simulink library "EV_ePWT"  (R2019b)
settings: Solver=VariableStepAuto  StartTime=0.0  StopTime=10.0  RelTol=1e-3
undefined symbols (not defined in the file): BTR, DiscIntNeverNeededParam, INV
libraries: simulink x1
(part 1 of 2)
Description:
  | User defined library for EV
settings Model: Creator=francesco.mantuano  LastModifiedBy=matteo.paganini

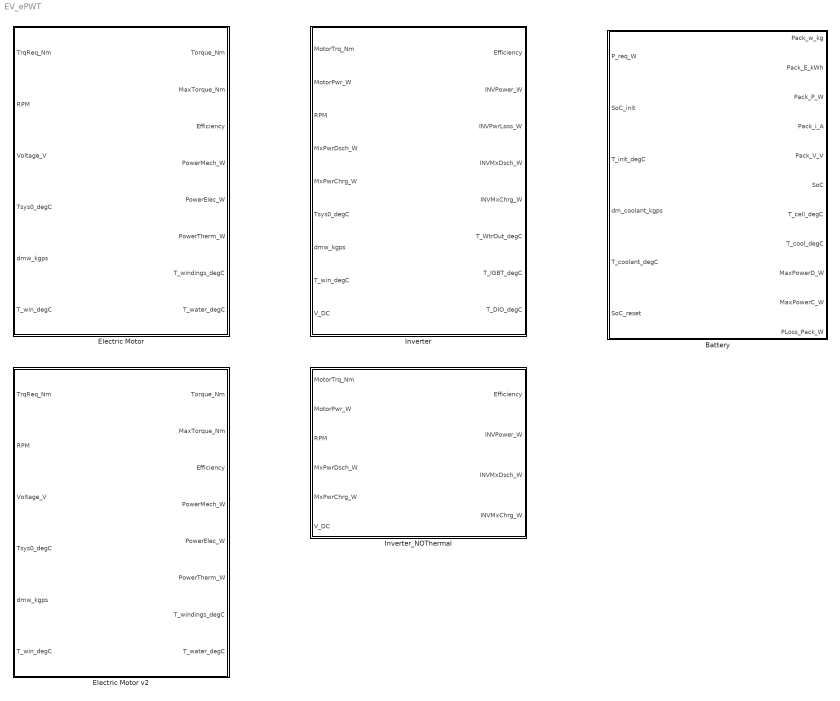
== system EV_ePWT ==
  Battery : Subsystem  mask(Battery 1RC){n_series=BTR.cell_p.n_series, n_parallel=BTR.cell_p.n_parallel, weight_ratio=0.7, C_cell_Ah=BTR.cell_p.capacity_nom, V_nominal=BTR.cell_p.voltage_nom, R_contact=0, V_low=BTR.cell_p.Vmin, V_up=BTR.cell_p.Vmax, R_th_KpW=BTR.cell_p.R_th, c_th=BTR.cell_p.c_th, weight=BTR.cell_p.weight, VoC_map=BTR.cell_p.VOC, VoC_SoC_bp=BTR.cell_p.SOC_bp_VOC, VoC_Temp_bp=BTR.cell_p.Temp_bp_VOC, VoC_C_bp=BTR.cell_p.C_bp, R0_map=BTR.cell_p.R0, R0_SoC_bp=BTR.cell_p.SOC_bp, R0_Temp_bp=BTR.cell_p.Temp_bp, R0_i_bp=BTR.cell_p.I_bp, R0_C_bp=BTR.cell_p.C_bp, R1_map=BTR.cell_p.R1, R1_SoC_bp=BTR.cell_p.SOC_bp, R1_Temp_bp=BTR.cell_p.Temp_bp, R1_i_bp=BTR.cell_p.I_bp, R1_C_bp=BTR.cell_p.C_bp, tau1_map=BTR.cell_p.tau, tau1_SoC_bp=BTR.cell_p.SOC_bp, tau1_Temp_bp=BTR.cell_p.Temp_bp, tau1_i_bp=BTR.cell_p.I_bp, tau1_C_bp=BTR.cell_p.C_bp, Limit_temp_bp=[-30 -10 0 55 57 58], Limit_map=[0 0.2 1 1 0.2 0], max_peak_crate=5, max_crate=2, peak_time=10}
      mask prompts: n_series "number of series"; n_parallel "number of parallel"; weight_ratio "cells/total weight ratio [-]"; C_cell_Ah "cell capacity [Ah]"; V_nominal "Nominal voltage [V]"; R_contact "R_contact [ohm]"; V_low "Voltage lower limit [V]"; V_up "Voltage upper limit [V]"; R_th_KpW "Thermal resistance [K/W]"; c_th "Specific heat capacity [J/(kgK)]"; weight "Cell weight [kg]"; VoC_map "Voltage map [V]"; VoC_SoC_bp "SoC breakpoints [-]"; VoC_Temp_bp "Temp breakpoints [degC]"; VoC_C_bp "C breakpoints [Ah]"; R0_map "R0 map [ohm]"; R0_SoC_bp "SoC breakpoints [-]"; R0_Temp_bp "Temp breakpoints [degC]"; R0_i_bp "i_cell breakpoints [A]"; R0_C_bp "C breakpoints [Ah]"; R1_map "R1 map [ohm]"; R1_SoC_bp "SoC breakpoints [-]"; R1_Temp_bp "Temp breakpoints [degC]"; R1_i_bp "i_cell breakpoints [A]"; R1_C_bp "C breakpoints [Ah]"; tau1_map "tau1 map [s]"; tau1_SoC_bp "SoC breakpoints [-]"; tau1_Temp_bp "Temp breakpoints [degC]"; tau1_i_bp "i_cell breakpoints [A]"; tau1_C_bp "C breakpoints [Ah]"; Limit_temp_bp "Limit Temp breakipoints [degC]"; Limit_map "Limit map [-]"; max_peak_crate "Max peak C-rate [1/h]"; max_crate "Max continuous C-rate [1/h]"; peak_time "C-rate peak time [s]"
      mask help:
      | 1RC battery model with simple BMS for c-rate, temperature and voltage limitations.
      | Includes simple thermal model and batery pack weights estimation
      mask DialogControl Container2 Prompt: Inputs description
      mask DialogControl DescTextVar Prompt: - P_req_W: power requested to battery [W] (negative is charge)
      mask DialogControl DescTextVar2 Prompt: - SoC_init: State of Charge initialization [-] (0 < SoC_init < 1)
      mask DialogControl DescTextVar3 Prompt: - T_init_degC: Cell temperature initialization [degC]
      mask DialogControl DescTextVar4 Prompt: - SoC_reset: reset of SoC (reset with falling to 0)
      mask DialogControl Container3 Prompt: Battery parameters
      mask DialogControl Container15 Prompt: Inputs
      mask DialogControl Container16 Prompt: Pack
      mask DialogControl Container17 Prompt: cell
      mask DialogControl Container20 Prompt: Thermals
      mask DialogControl Container9 Prompt: Cell properties
      mask DialogControl Container10 Prompt: Voltage f(SoC,Temp,C)
      mask DialogControl Container11 Prompt: R0 f(SoC,Temp,i_cell,C)
      mask DialogControl Container12 Prompt: R1 f(SoC,Temp,i_cell,C)
      mask DialogControl Container13 Prompt: tau1 f(SoC,Temp,i_cell,C)
      mask DialogControl Container18 Prompt: SOF
      mask DialogControl Container22 Prompt: Temperature limitation
      mask DialogControl Container23 Prompt: C-rate limitation
  Electric Motor : Subsystem  mask(Motor){Mass_w=1, cp_w=385, Mass_s=1, cp_s=385, ThrmRtos=0.005, ThrmRtow=0.005, MaxT=180, RPM_bp1=0, voltage_bp=0, Torque_map=0, RPM_bp2=0, torque_bp=0, temp_bp=0, Efficiency_map=0}
      mask prompts: Mass_w "Windings Mass [kg]"; cp_w "Windings cp [J/(kg*K)]"; Mass_s "Stator Mass [kg]"; cp_s "Stator av. cp [J/(kg*K)]"; ThrmRtos "Thermal resistance 1 [K/W]"; ThrmRtow "Thermal resistance 2 [K/W]"; MaxT "Max temperature [degC] allowed"; RPM_bp1 "RPM breakpoints"; voltage_bp "Voltage [V] breakpoints"; Torque_map "Torque map [Nm]"; RPM_bp2 "RPM breakpoints"; torque_bp "Torque [Nm] breakpoints"; temp_bp "Temperature [degC] breakpoints"; Efficiency_map "Efficiency map [-]"
      mask help:
      | The Motor block is a map based block. It has as output the limited torque, power and efficiency.
      | It also includes a thermal model that outputs the motor and cooling liquid temperature.
      |
      | The inputs required are the torque(RPM, V) and efficiency(RPM, Trq, Temp) maps. The derating is thermal; the windings temperature is calculated taking into account the thermal capacity [J/K] and the thermal resistance [K/W]. "Thermal resistance 1" is the one between the windings and the stator, "Thermal resistance 2" is the one between the stator and the liquid cooling (constant with massflow).
      mask DialogControl Container2 Prompt: Input signals description
      mask DialogControl DescTextVar Prompt: - TrqReq_Nm: torque requested [Nm]
      mask DialogControl Control3 Prompt: - RPM: actual RPM of the motor
      mask DialogControl Control6 Prompt: - Voltage_V: voltage of the Inverter [V]
      mask DialogControl Control4 Prompt: - Tsys0_degC: initial temperature of the system [degC]
      mask DialogControl Control5 Prompt: - dmw_kgps: mass flow of the cooling liquid [kg/s]
      mask DialogControl Control7 Prompt: - T_win_degC: liquid cooling inlet temperature [degC]
      mask DialogControl Container3 Prompt: Motor parameters
      mask DialogControl Container9 Prompt: Constants
      mask DialogControl Container5 Prompt: Torque map
      mask DialogControl Container5_copy Prompt: Efficiency map
  Electric Motor v2 : Subsystem  mask(Motor){Mass_w=1, cp_w=385, Mass_s=1, cp_s=385, ThrmRtos=0.005, MaxT=180, RPM_bp1=0, voltage_bp=0, Torque_map=0, RPM_bp2=0, torque_bp=0, temp_bp=0, Efficiency_map=0, PL_torque_bp=-250:50:250, PL_RPM_bp=1000:1000:15000, PL_V_bp=450:100:750, PL_map=ones(11,15,4)*200, D_h=13.33e-3, A_n=2e-4, lpm_tar=10, R_tar=0.0154, thermal_mode=from efficiency maps}
      mask prompts: Mass_w "Windings Mass [kg]"; cp_w "Windings cp [J/(kg*K)]"; Mass_s "Stator Mass [kg]"; cp_s "Stator av. cp [J/(kg*K)]"; ThrmRtos "Thermal resistance 1 [K/W]"; MaxT "Max temperature [degC] allowed"; RPM_bp1 "RPM breakpoints"; voltage_bp "Voltage [V] breakpoints"; Torque_map "Torque map [Nm]"; RPM_bp2 "RPM breakpoints"; torque_bp "Torque [Nm] breakpoints"; temp_bp "Temperature [degC] breakpoints"; Efficiency_map "Efficiency map [-]"; PL_torque_bp "Torque [Nm] breakpoints"; PL_RPM_bp "RPM breakpoints"; PL_V_bp "V_DC [V] breakpoints"; PL_map "Power losses map [W]"; D_h "Hydraulic diameter [m]"; A_n "Normal surface [sm]"; lpm_tar "Refernce flowrate [lpm]"; R_tar "Target R_th @lpm_ref"; thermal_mode "Thermal losses calculation"
      mask help:
      | The Motor block is a map based block. It has as output the limited torque, power and efficiency.
      | It also includes a thermal model that outputs the motor and cooling liquid temperature.
      |
      | The inputs required are the torque(RPM, V) and efficiency(RPM, Trq, Temp) maps. The derating is thermal; the windings temperature is calculated taking into account the thermal capacity [J/K] and the thermal resistance [K/W]. "Thermal resistance 1" is the one between the windings and the stator, the thermal resistance between the stator and the liquid cooling is calculated with Dittus-Boelter correlation (open block to inspect the formula).
      mask TypeOptions thermal_mode: from efficiency maps | from power losses maps
      mask DialogControl Container2 Prompt: Input signals description
      mask DialogControl DescTextVar Prompt: - TrqReq_Nm: torque requested [Nm]
      mask DialogControl Control3 Prompt: - RPM: actual RPM of the motor
      mask DialogControl Control6 Prompt: - Voltage_V: voltage of the Inverter [V]
      mask DialogControl Control4 Prompt: - Tsys0_degC: initial temperature of the system [degC]
      mask DialogControl Control5 Prompt: - dmw_kgps: mass flow of the cooling liquid [kg/s]
      mask DialogControl Control7 Prompt: - T_win_degC: liquid cooling inlet temperature [degC]
      mask DialogControl Container3 Prompt: Motor parameters
      mask DialogControl Container9 Prompt: Constants
      mask DialogControl Container5 Prompt: Torque map
      mask DialogControl Container5_copy Prompt: Efficiency map
      mask DialogControl Container5_copy_copy_copy Prompt: Power losses map
      mask DialogControl Container5_copy_copy Prompt: Cooling (geometrical data)
  Inverter : Subsystem  mask(Inverter){C_IGBT=45, R_IGBT=0.038, C_DIO=10, R_DIO=0.070, C_HS=200, R_TIM=0.021, cp_cool=3140, n_poles=6, V_DC_ref=730, RPM_bp=1000:1000:15000, torque_bp=-250:50:250, Efficiency_map=ones(15,11)*0.95, PL_torque_bp=-250:50:250, PL_RPM_bp=1000:1000:15000, PL_V_bp=450:100:750, PL_map=ones(11,15,4)*200, thermal_mode=from efficiency maps}
      mask prompts: C_IGBT "Heat capacity [J/K]"; R_IGBT "Thermal resistance [K/W]"; C_DIO "Heat capacity [J/K]"; R_DIO "Thermal resistance [K/W]"; C_HS "HS Heat capacity [J/K]"; R_TIM "TIM Thermal resistance [K/W]"; cp_cool "cp water-glycol 50-50"; n_poles "number of pole pairs"; RPM_bp "RPM breakpoints"; torque_bp "Torque [Nm] breakpoints"; Efficiency_map "Efficiency map [-]"; PL_torque_bp "Torque [Nm] breakpoints"; PL_RPM_bp "RPM breakpoints"; PL_V_bp "V_DC [V] breakpoints"; PL_map "Power losses map [W]"; thermal_mode "Thermal losses calculation"
      mask help:
      | The Inverter block is a map based block. It has as output the efficiency, power and max deliverable power.
      | It also includes a thermal model that outputs the IGBT, Diode and cooling liquid temperature.
      mask TypeOptions thermal_mode: from efficiency maps | from power losses maps
      mask DialogControl Container2 Prompt: Inputs description
      mask DialogControl DescTextVar Prompt: - MotorTrq_Nm: motor torque [Nm]
      mask DialogControl DescTextVar_copy Prompt: - MotorPwr_W: motor electric power [W]
      mask DialogControl Control3 Prompt: - RPM: actual RPM of the motor
      mask DialogControl Control6 Prompt: - MxPwrDsch_W: max DC discharge deliverable power [W]
      mask DialogControl Control6_copy Prompt: - MxPwrChrg_W: max DC charge deliverable power [W]
      mask DialogControl Control4 Prompt: - Tsys0_degC: initial temperature of the system [degC]
      mask DialogControl Control5 Prompt: - dmw_kgps: mass flow of the cooling liquid [kg/s]
      mask DialogControl Control7 Prompt: - T_win_degC: liquid cooling inlet temperature [degC]
      mask DialogControl Container3 Prompt: Inverter parameters
      mask DialogControl Container9 Prompt: Constants
      mask DialogControl Container10 Prompt: IGBT
      mask DialogControl Container10_copy Prompt: DIODE
      mask DialogControl Container10_copy_copy Prompt: OTHER
      mask DialogControl Container5_copy Prompt: Efficiency map
      mask DialogControl Container5_copy_copy Prompt: Power losses map
  Inverter_NOThermal : Subsystem  mask(Inverter){RPM_bp=INV.Front.bp_RPM_Mtr, torque_bp=INV.Front.bp_Torque_Nm_Mtr, Efficiency_map=INV.Front.Eff_Table_r}
      mask prompts: RPM_bp "RPM breakpoints"; torque_bp "Torque [Nm] breakpoints"; Efficiency_map "Efficiency map [-]"
      mask help: The Inverter block is a map based block. It has as output the efficiency, power and max deliverable power.
      mask DialogControl Container2 Prompt: Inputs description
      mask DialogControl DescTextVar Prompt: - MotorTrq_Nm: motor torque [Nm]
      mask DialogControl DescTextVar_copy Prompt: - MotorPwr_W: motor electric power [W]
      mask DialogControl Control3 Prompt: - RPM: actual RPM of the motor
      mask DialogControl Control6 Prompt: - MxPwrDsch_W: max DC discharge deliverable power [W]
      mask DialogControl Control6_copy Prompt: - MxPwrChrg_W: max DC charge deliverable power [W]
      mask DialogControl Container3 Prompt: Inverter parameters
      mask DialogControl Container5_copy Prompt: Efficiency map

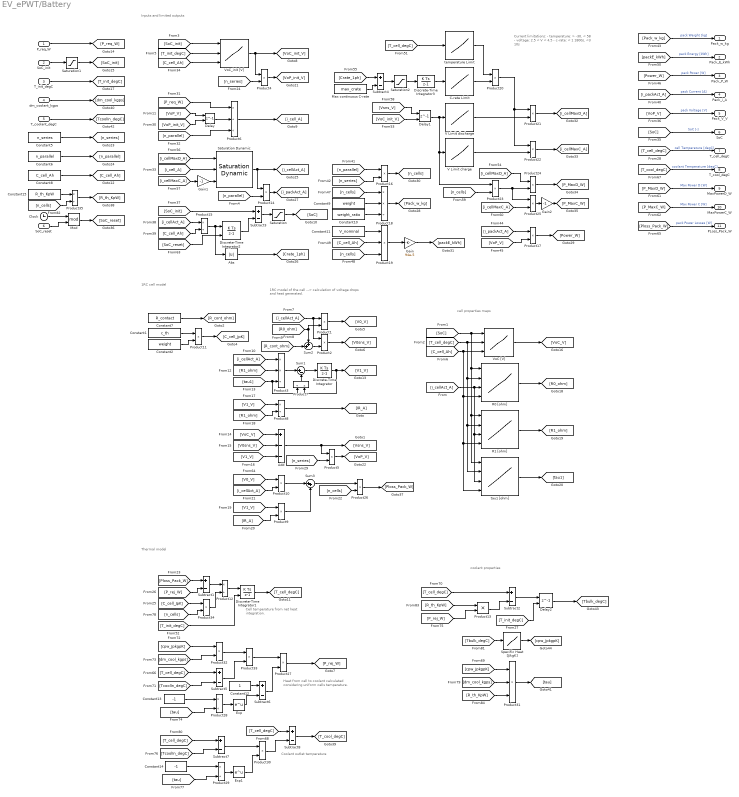
== system EV_ePWT/Battery ==
  note: 1RC model of the cell --> calculation of voltage drops and heat generated.
  note: cell properties maps
  note: Current limitations:
      | - temperature: > -30, < 58
      | - voltage: 2.5 < V < 4.5
      | - c-rate: < 1 1800s, <3 10s
  note: Inputs and limited outputs
  note: 1RC cell model
  note: Heat from cell to coolant calculated considering uniform cells temperature.
  note: Thermal model
  note: Cell temperature from net heat integration.
  note: Coolant outlet temperature
  note: coolant properties
  P_req_W : Inport
  SoC_init : Inport  Port=2
  T_init_degC : Inport  Port=3
  dm_coolant_kgps : Inport  Port=4
  T_coolant_degC : Inport  Port=5
  SoC_reset : Inport  Port=6
  Abs : Abs
  Add : Sum  Inputs=+--
  C-rate Limit : Lookup_n-D  NumberOfTableDimensions=1  BreakpointsForDimension1=[0 peak_time 60]  BreakpointsForDimension2=BTR.cell_p.Temp_bp_VOC  BreakpointsForDimension3=BTR.cell_p.C_bp  Table=[max_peak_crate max_peak_crate max_crate]*C_cell_Ah  ExtrapMethod=Clip  InternalRulePriority=Speed  RndMeth=Simplest  InputSameDT=on
  Clock : Clock
  Constant1 : Constant  Value=c_th
  Constant10 : Constant  Value=weight_ratio
  Constant11 : Constant  Value=V_nominal
  Constant12 : Constant
  Constant13 : Constant  Value=-1
  Constant14 : Constant  Value=-1
  Constant15 : Constant  Value=R_th_KpW
  Constant2 : Constant  Value=weight
  Constant5 : Constant  Value=n_series
  Constant6 : Constant  Value=n_parallel
  Constant7 : Constant  Value=R_contact
  Constant8 : Constant  Value=C_cell_Ah
  Constant9 : Constant  Value=weight
  Delay : Delay  DelayLength=1  InitialConditionSource=Input port
      settings: InputPortMap=u0,p4
  Delay1 : Delay  DelayLength=1  InitialConditionSource=Input port
      settings: InputPortMap=u0,p4
  Delay2 : Delay  DelayLength=1  InitialConditionSource=Input port
      settings: InputPortMap=u0,p4
  Discrete-Time Integrator : DiscreteIntegrator  SampleTime=-1  ICPrevOutput=DiscIntNeverNeededParam  ICPrevScaledInput=DiscIntNeverNeededParam
  Discrete-Time Integrator1 : DiscreteIntegrator  InitialConditionSource=external  SampleTime=-1  ICPrevOutput=DiscIntNeverNeededParam  ICPrevScaledInput=DiscIntNeverNeededParam
  Discrete-Time Integrator2 : DiscreteIntegrator  gainval=1/3600  ExternalReset=falling  SampleTime=-1  UpperSaturationLimit=1  LowerSaturationLimit=0  ICPrevOutput=DiscIntNeverNeededParam  ICPrevScaledInput=DiscIntNeverNeededParam
  Discrete-Time Integrator3 : DiscreteIntegrator  gainval=1  SampleTime=-1  LimitOutput=on  LowerSaturationLimit=0  ICPrevOutput=DiscIntNeverNeededParam  ICPrevScaledInput=DiscIntNeverNeededParam
  Exp : Math  SignedPower=off  SaturateOnIntegerOverflow=on
  Exp1 : Math  SignedPower=off  SaturateOnIntegerOverflow=on
  Gain : Gain  Gain=94e-5
  Gain1 : Gain  Gain=-1
  Gain2 : Gain  Gain=-1
  Max continuous C-rate : Constant  Value=max_crate
  Mod : Math  Operator=mod  SignedPower=off  SaturateOnIntegerOverflow=on
  Product{1..2,4..5,11,13..14,16..17,20..27,30,32..34} (21 alike) : Product
  Product10 : Product  Inputs=**
  Product{8,12,15,28..29,35} (6 alike) : Product  Inputs=*/
  Product18 : Product  Inputs=**/
  Product19 : Product  Inputs=***
  Product3 : Product  Inputs=**/
  Product31 : Product  Inputs=3
  Product6 : Product  Inputs=*//
  Product7 : Product  Inputs=/*
  Product9 : Product  Inputs=**
  R0 [ohm] : Lookup_n-D  NumberOfTableDimensions=4  BreakpointsForDimension1=R0_SoC_bp  BreakpointsForDimension2=R0_Temp_bp  BreakpointsForDimension3=R0_i_bp  BreakpointsForDimension4=R0_C_bp  Table=R0_map  ExtrapMethod=Clip  InternalRulePriority=Speed  RndMeth=Simplest  InputSameDT=on
  R1 [ohm] : Lookup_n-D  NumberOfTableDimensions=4  BreakpointsForDimension1=R1_SoC_bp  BreakpointsForDimension2=R1_Temp_bp  BreakpointsForDimension3=R1_i_bp  BreakpointsForDimension4=R1_C_bp  Table=R1_map  ExtrapMethod=Clip  InternalRulePriority=Speed  RndMeth=Simplest  InputSameDT=on
  Saturation : Saturate  UpperLimit=1  LowerLimit=0
  Saturation Dynamic : simulink/Discontinuities/Saturation Dynamic  OutMin=[]  OutMax=[]  OutDataTypeStr=Inherit: Same as second input  OutDataType=fixdt(1, 16)  OutScaling=2^-10  DoSatur=off
  Saturation1 : Saturate  UpperLimit=1  LowerLimit=0
  Saturation2 : Saturate  UpperLimit=1  LowerLimit=-1
  Specific Heat [J/kgK] : Lookup_n-D  NumberOfTableDimensions=1  BreakpointsForDimension1=[-45.56 -17.78 10 37.77 65.55 93.33 121.11 148.88 176.66]  Table=[3841.6,3888.1,3934.6,3981.1,4027.6,4074.0,4120.5,4167.0,4213.6]  ExtrapMethod=Clip  RndMeth=Simplest  InputSameDT=on
  Subtract{1..8} (8 alike) : Sum  Inputs=+-
  Sum1 : Sum  Inputs=|+-
  Sum2 : Sum  Inputs=++|
  Sum3 : Sum  Inputs=|++
  V Limit charge : Lookup_n-D  NumberOfTableDimensions=1  BreakpointsForDimension1=[V_low V_up-0.2 V_up]  BreakpointsForDimension2=BTR.cell_p.Temp_bp_VOC  BreakpointsForDimension3=BTR.cell_p.C_bp  Table=[1 1 0]  ExtrapMethod=Clip  InternalRulePriority=Speed  RndMeth=Simplest  InputSameDT=on
  V Limit discharge : Lookup_n-D  NumberOfTableDimensions=1  BreakpointsForDimension1=[V_low V_low+0.2 V_up]  BreakpointsForDimension2=BTR.cell_p.Temp_bp_VOC  BreakpointsForDimension3=BTR.cell_p.C_bp  Table=[0 1 1]  ExtrapMethod=Clip  InternalRulePriority=Speed  RndMeth=Simplest  InputSameDT=on
  VoC [V] : Lookup_n-D  NumberOfTableDimensions=3  BreakpointsForDimension1=VoC_SoC_bp  BreakpointsForDimension2=VoC_Temp_bp  BreakpointsForDimension3=VoC_C_bp  Table=VoC_map  ExtrapMethod=Clip  InternalRulePriority=Speed  RndMeth=Simplest  InputSameDT=on
  VoC_init [V] : Lookup_n-D  NumberOfTableDimensions=3  BreakpointsForDimension1=BTR.cell_p.SOC_bp_VOC  BreakpointsForDimension2=BTR.cell_p.Temp_bp_VOC  BreakpointsForDimension3=BTR.cell_p.C_bp  Table=BTR.cell_p.VOC  ExtrapMethod=Clip  InternalRulePriority=Speed  RndMeth=Simplest  InputSameDT=on
  tau1 [ohm] : Lookup_n-D  NumberOfTableDimensions=4  BreakpointsForDimension1=tau1_SoC_bp  BreakpointsForDimension2=tau1_Temp_bp  BreakpointsForDimension3=tau1_i_bp  BreakpointsForDimension4=tau1_C_bp  Table=tau1_map  ExtrapMethod=Clip  InternalRulePriority=Speed  RndMeth=Simplest  InputSameDT=on
  temperature Limit : Lookup_n-D  NumberOfTableDimensions=1  BreakpointsForDimension1=Limit_temp_bp  BreakpointsForDimension2=BTR.cell_p.Temp_bp_VOC  BreakpointsForDimension3=BTR.cell_p.C_bp  Table=Limit_map  ExtrapMethod=Clip  InternalRulePriority=Speed  RndMeth=Simplest  InputSameDT=on
  Pack_w_kg : Outport
  Pack_E_kWh : Outport  Port=2
  Pack_P_W : Outport  Port=3
  Pack_i_A : Outport  Port=4
  Pack_V_V : Outport  Port=5
  SoC : Outport  Port=6
  T_cell_degC : Outport  Port=7
  T_cool_degC : Outport  Port=8
  MaxPowerD_W : Outport  Port=9
  MaxPowerC_W : Outport  Port=10
  PLoss_Pack_W : Outport  Port=11
  wires:
  Product1/1 -> [V0_V]
  [i_cellAct_A] -> Product1/1, Product2/1
  [R0_ohm] -> Sum2/1, Product1/2
  [R_cont_ohm] -> Sum2/2
  Sum2/1 -> Product2/2
  R0 [ohm]/1 -> [R0_ohm]
  VoC [V]/1 -> [VoC_V]
  SoC_init/1 -> Saturation1/1
  T_init_degC/1 -> [T_init_degC]
  P_req_W/1 -> [P_req_W]
  tau1 [ohm]/1 -> [tau1]
  R1 [ohm]/1 -> [R1_ohm]
  [SoC] -> tau1 [ohm]/1, R1 [ohm]/1, R0 [ohm]/1, VoC [V]/1
  [T_cell_degC] -> tau1 [ohm]/2, R1 [ohm]/2, R0 [ohm]/2, VoC [V]/2
  [C_cell_Ah] -> tau1 [ohm]/4, R1 [ohm]/4, R0 [ohm]/4, VoC [V]/3
  [i_cellAct_A] -> tau1 [ohm]/3, R1 [ohm]/3, R0 [ohm]/3
  Constant7/1 -> [R_cont_ohm]
  Product2/1 -> [V0sns_V]
  Discrete-Time Integrator/1 -> Product7/2, [V1_V]
  Sum1/1 -> Discrete-Time Integrator/1
  Product3/1 -> Sum1/1
  [i_cellAct_A] -> Product3/1
  [R1_ohm] -> Product3/2
  [tau1] -> Product7/1, Product3/3
  Product7/1 -> Sum1/2
  [VoC_V] -> Add/1
  [V0sns_V] -> Add/2
  [V1_V] -> Add/3
  Add/1 -> Product5/1, [Vsns_V]
  [V1_V] -> Product8/1
  [R1_ohm] -> Product8/2
  Product8/1 -> [IR_A]
  [V1_V] -> Product9/1
  [IR_A] -> Product9/2
  [i_cellAct_A] -> Product10/2
  [V0_V] -> Product10/1
  Product9/1 -> Sum3/2
  Product10/1 -> Sum3/1
  Sum3/1 -> Product26/1
  Constant1/1 -> Product11/1
  Constant2/1 -> Product11/2
  Product11/1 -> [C_cell_JpK]
  [Ploss_Pack_W] -> Subtract1/1
  [P_rej_W] -> Subtract1/2
  Subtract1/1 -> Product12/1
  Product12/1 -> Discrete-Time Integrator1/1
  Discrete-Time Integrator1/1 -> [T_cell_degC]
  [T_cell_degC] -> T_cell_degC/1  "cell Temperature [degC]"
  VoC_init [V]/1 -> [VoC_init_V], Product4/1
  [SoC_init] -> VoC_init [V]/1
  [T_init_degC] -> VoC_init [V]/2
  Product4/1 -> [VoP_init_V]
  Constant5/1 -> [n_series]
  Constant6/1 -> [n_parallel]
  [n_series] -> Product4/2
  [n_series] -> Product5/2
  Product5/1 -> [VoP_V]
  Constant8/1 -> [C_cell_Ah]
  [VoP_init_V] -> Delay/2
  [VoP_V] -> Delay/1
  Delay/1 -> Product6/2
  [n_parallel] -> Product6/3
  [P_req_W] -> Product6/1
  Product6/1 -> [i_cell_A]
  [C_cell_Ah] -> VoC_init [V]/3
  Saturation Dynamic/1 -> Product14/1, [i_cellAct_A]
  [i_cell_A] -> Saturation Dynamic/2
  [SoC_init] -> Subtract3/1
  Subtract3/1 -> Saturation/1
  Discrete-Time Integrator2/1 -> Subtract3/2
  Product15/1 -> Discrete-Time Integrator2/1, Abs/1
  [i_cellAct_A] -> Product15/1
  [C_cell_Ah] -> Product15/2
  [SoC] -> SoC/1  "SoC [-]"
  [VoP_V] -> Pack_V_V/1  "pack Voltage [V]"
  [n_parallel] -> Product14/2
  Product14/1 -> [i_packAct_A]
  [n_parallel] -> Product16/1
  [i_packAct_A] -> Product17/1
  [VoP_V] -> Product17/2
  Product17/1 -> [Power_W]
  [Pack_w_kg] -> Pack_w_kg/1  "pack Weight [kg]"
  [n_series] -> Product16/2
  Product16/1 -> [n_cells]
  Constant11/1 -> Product19/1
  [C_cell_Ah] -> Product19/2
  [n_cells] -> Product19/3
  Product19/1 -> Gain/1
  Gain/1 -> [packE_kWh]
  [packE_kWh] -> Pack_E_kWh/1  "pack Energy [kWh]"
  [Power_W] -> Pack_P_W/1  "pack Power [W]"
  [i_packAct_A] -> Pack_i_A/1  "pack Current [A]"
  [n_cells] -> Product18/1
  Constant9/1 -> Product18/2
  Constant10/1 -> Product18/3
  Product18/1 -> [Pack_w_kg]
  [T_init_degC] -> Discrete-Time Integrator1/2
  [T_cell_degC] -> temperature Limit/1
  [Vsns_V] -> Delay1/1
  [VoC_init_V] -> Delay1/2
  Delay1/1 -> Product23/1, V Limit charge/1, V Limit discharge/1
  Abs/1 -> [Crate_1ph]
  [Crate_1ph] -> Subtract4/1
  Max continuous C-rate/1 -> Subtract4/2
  Subtract4/1 -> Saturation2/1
  Saturation/1 -> [SoC]
  Discrete-Time Integrator3/1 -> C-rate Limit/1
  C-rate Limit/1 -> Product20/2
  temperature Limit/1 -> Product20/1
  V Limit discharge/1 -> Product21/2
  V Limit charge/1 -> Product22/2
  Product20/1 -> Product22/1, Product21/1
  Product21/1 -> [i_cellMaxD_A]
  Product22/1 -> [i_cellMaxC_A]
  [i_cellMaxC_A] -> Gain1/1
  [i_cellMaxD_A] -> Saturation Dynamic/1
  Gain1/1 -> Saturation Dynamic/3
  [n_cells] -> Product23/2
  Product24/1 -> [P_MaxD_W]
  Product23/1 -> Product25/1, Product24/2
  [i_cellMaxD_A] -> Product24/1
  [i_cellMaxC_A] -> Product25/2
  [P_MaxC_W] -> MaxPowerC_W/1  "Max Power C [W]"
  [P_MaxD_W] -> MaxPowerD_W/1  "Max Power D [W]"
  Product25/1 -> Gain2/1
  Gain2/1 -> [P_MaxC_W]
  Saturation1/1 -> [SoC_init]
  Saturation2/1 -> Discrete-Time Integrator3/1
  [SoC_reset] -> Discrete-Time Integrator2/2
  [n_cells] -> Product26/2
  Product26/1 -> [Ploss_Pack_W]
  [Ploss_Pack_W] -> PLoss_Pack_W/1  "pack Power Losses [W]"
  dm_coolant_kgps/1 -> [dm_cool_kgps]
  [T_cool_degC] -> T_cool_degC/1  "coolant Temperature [degC]"
  Constant12/1 -> Subtract6/1
  Product28/1 -> Exp/1
  [tau] -> Product28/2
  Product29/1 -> Exp1/1
  [TcoolIn_degC] -> Subtract5/2
  Subtract6/1 -> Product27/2
  Product30/1 -> Subtract8/2
  [dm_cool_kgps] -> Product32/2
  [R_th_KpW] -> Product31/3
  [cpw_JpkgpK] -> Product31/1
  Subtract8/1 -> [T_cool_degC]
  Subtract7/1 -> Product30/1
  [T_cell_degC] -> Subtract5/1
  Product33/1 -> Product27/1
  [T_cell_degC] -> Subtract8/1
  Product27/1 -> [P_rej_W]
  Constant14/1 -> Product29/1
  [dm_cool_kgps] -> Product31/2
  Exp1/1 -> Product30/2
  [tau] -> Product29/2
  [T_cell_degC] -> Subtract7/1
  [TcoolIn_degC] -> Subtract7/2
  Product31/1 -> [tau]
  Constant13/1 -> Product28/1
  Exp/1 -> Subtract6/2
  Subtract5/1 -> Product33/2
  Product32/1 -> Product33/1
  T_coolant_degC/1 -> [TcoolIn_degC]
  [cpw_JpkgpK] -> Product32/1
  [P_rej_W] -> Product13/2
  Subtract2/1 -> Delay2/1
  [R_th_KpW] -> Product13/1
  Delay2/1 -> [Tbulk_degC]
  [T_cell_degC] -> Subtract2/1
  Product13/1 -> Subtract2/2
  [T_init_degC] -> Delay2/2
  Specific Heat [J/kgK]/1 -> [cpw_JpkgpK]
  [Tbulk_degC] -> Specific Heat [J/kgK]/1
  [C_cell_JpK] -> Product34/1
  [n_cells] -> Product34/2
  Product34/1 -> Product12/2
  Constant15/1 -> Product35/1
  [n_cells] -> Product35/2
  Product35/1 -> [R_th_KpW]
  Clock/1 -> Mod/1
  Mod/1 -> [SoC_reset]
  SoC_reset/1 -> Mod/2

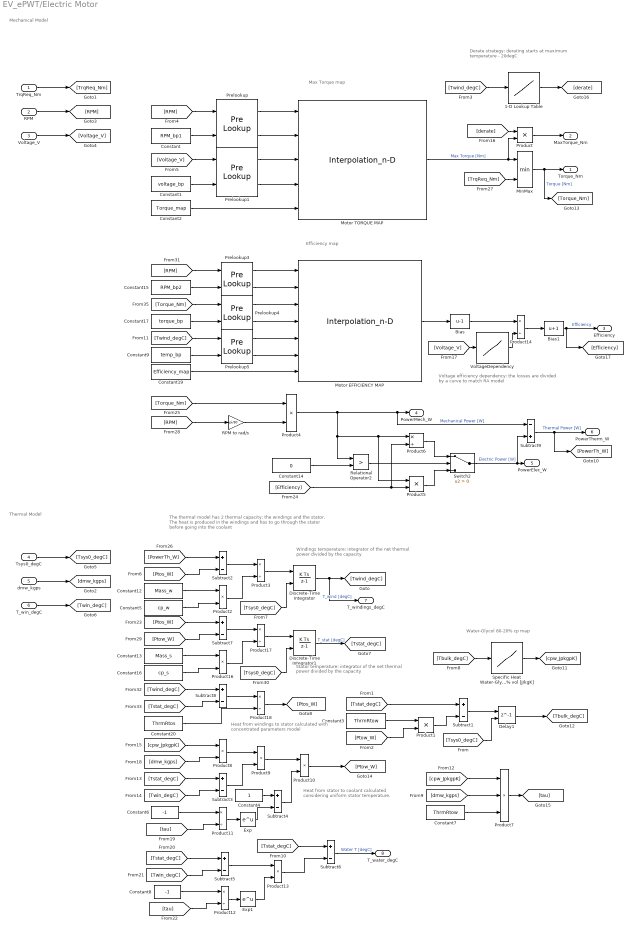
== system EV_ePWT/Electric Motor ==
  note: Mechanical Model
  note: Thermal Model
  note: Max Torque map
  note: Efficiency map
  note: Derate strategy: derating starts at maximum temperature - 20degC
  note: Voltage efficiency dependency: the losses are divided by a curve to match RA model
  note: Water-Glycol 80-20% cp map
  note: The thermal model has 2 thermal capacity: the windings and the stator. The heat is produced in the windings and has to go through the stator before going into the coolant
  note: Windings temperature: integrator of the net thermal power divided by the capacity
  note: Stator temperature: integrator of the net thermal power divided by the capacity
  note: Heat from windings to stator calculated with concentrated parameters model
  note: Heat from stator to coolant calculated considering uniform stator temperature.
  TrqReq_Nm : Inport
  RPM : Inport  Port=2
  Voltage_V : Inport  Port=3
  Tsys0_degC : Inport  Port=4
  dmw_kgps : Inport  Port=5
  T_win_degC : Inport  Port=6
  1-D Lookup Table : Lookup_n-D  NumberOfTableDimensions=1  BreakpointsForDimension1=[-20 80 (MaxT-20) MaxT]  Table=[1 1 1 0]  InternalRulePriority=Speed  RndMeth=Simplest  InputSameDT=on
  Bias : Bias  Bias=-1
  Bias1 : Bias  Bias=1
  Constant : Constant  Value=RPM_bp1
  Constant1 : Constant  Value=voltage_bp
  Constant12 : Constant  Value=Mass_w
  Constant13 : Constant  Value=Mass_s
  Constant14 : Constant  Value=0
  Constant15 : Constant  Value=RPM_bp2
  Constant16 : Constant  Value=cp_s
  Constant17 : Constant  Value=torque_bp
  Constant19 : Constant  Value=Efficiency_map
  Constant2 : Constant  Value=Torque_map
  Constant20 : Constant  Value=ThrmRtos
  Constant3 : Constant  Value=ThrmRtow
  Constant4 : Constant
  Constant5 : Constant  Value=cp_w
  Constant6 : Constant  Value=-1
  Constant7 : Constant  Value=ThrmRtow
  Constant8 : Constant  Value=-1
  Constant9 : Constant  Value=temp_bp
  Delay1 : Delay  DelayLength=1  InitialConditionSource=Input port
      settings: InputPortMap=u0,p4
  Discrete-Time Integrator : DiscreteIntegrator  InitialConditionSource=external  SampleTime=-1  ICPrevOutput=DiscIntNeverNeededParam  ICPrevScaledInput=DiscIntNeverNeededParam
  Discrete-Time Integrator1 : DiscreteIntegrator  InitialConditionSource=external  SampleTime=-1  ICPrevOutput=DiscIntNeverNeededParam  ICPrevScaledInput=DiscIntNeverNeededParam
  Exp : Math  SignedPower=off  SaturateOnIntegerOverflow=on
  Exp1 : Math  SignedPower=off  SaturateOnIntegerOverflow=on
  MinMax : MinMax  Inputs=2
  Motor EFFICIENCY MAP : Interpolation_n-D  NumberOfTableDimensions=3  TableSource=Input port
      settings: InputPortMap=u0,u1,u2,u3,u4,u5,p2
  Motor TORQUE MAP : Interpolation_n-D  TableSource=Input port
      settings: InputPortMap=u0,u1,u2,u3,p2
  Prelookup{,3..5} (4 alike) : PreLookup  BreakpointsDataSource=Input port  BreakpointsData=[1:4]  FractionDataTypeStr=double
      settings: InputPortMap=u0,p1
  Prelookup1 : PreLookup  BreakpointsDataSource=Input port  BreakpointsData=[1:4]  ExtrapMethod=Linear  FractionDataTypeStr=double
      settings: InputPortMap=u0,p1
  Product{,1..2,4..5,8..10,13,16} (10 alike) : Product
  Product{3,6,11..12,14,17..18} (7 alike) : Product  Inputs=*/
  Product7 : Product  Inputs=3
  RPM to rad/s : Gain  Gain=pi/30
  Relational Operator2 : RelationalOperator  Operator=>  OutDataTypeStr=boolean  RndMeth=Simplest
  Specific Heat Water-Glycol 80-20% vol [J/kgK] : Lookup_n-D  NumberOfTableDimensions=1  BreakpointsForDimension1=[-45.56 -17.78 10 37.77 65.55 93.33 121.11 148.88 176.66]  Table="[3841.6 3888.1  3934.6 3981.1 4027.6 4074.0 4120.5 4167.0 4213.6]"  ExtrapMethod=Clip  RndMeth=Simplest  InputSameDT=on
  Subtract{1..8} (8 alike) : Sum  Inputs=+-
  Subtract9 : Sum  Inputs=-+
  Switch2 : Switch  Criteria=u2 > Threshold
  VoltageDependency : Lookup_n-D  NumberOfTableDimensions=1  BreakpointsForDimension1=430:25:730  Table=1-exp(-(430:25:730)/73)*200  InternalRulePriority=Speed  RndMeth=Simplest  InputSameDT=on
  Torque_Nm : Outport
  MaxTorque_Nm : Outport  Port=2
  Efficiency : Outport  Port=3
  PowerMech_W : Outport  Port=4
  PowerElec_W : Outport  Port=5
  PowerTherm_W : Outport  Port=6
  T_windings_degC : Outport  Port=7
  T_water_degC : Outport  Port=8
  wires:
  Constant1/1 -> Prelookup1/2
  [RPM] -> Prelookup/1
  Prelookup/1 -> Motor TORQUE MAP/1
  [Voltage_V] -> Prelookup1/1
  Prelookup1/2 -> Motor TORQUE MAP/4
  RPM/1 -> [RPM]
  Prelookup1/1 -> Motor TORQUE MAP/3
  Voltage_V/1 -> [Voltage_V]
  Tsys0_degC/1 -> [Tsys0_degC]
  Prelookup/2 -> Motor TORQUE MAP/2
  TrqReq_Nm/1 -> [TrqReq_Nm]
  Constant/1 -> Prelookup/2
  Constant2/1 -> Motor TORQUE MAP/5
  Motor TORQUE MAP/1 -> Product/2, MinMax/1  "Max Torque [Nm]"
  [TrqReq_Nm] -> MinMax/2
  MinMax/1 -> [Torque_Nm], Torque_Nm/1  "Torque [Nm]"
  Motor EFFICIENCY MAP/1 -> Bias/1
  Constant15/1 -> Prelookup3/2
  Prelookup3/2 -> Motor EFFICIENCY MAP/2
  [Torque_Nm] -> Prelookup4/1
  Prelookup3/1 -> Motor EFFICIENCY MAP/1
  [RPM] -> Prelookup3/1
  Constant17/1 -> Prelookup4/2
  [RPM] -> RPM to rad/s/1
  [Torque_Nm] -> Product4/1
  RPM to rad/s/1 -> Product4/2
  Product4/1 -> Product5/1, Product6/1, Relational Operator2/1, Subtract9/1, PowerMech_W/1  "Mechanical Power [W]"
  Constant14/1 -> Relational Operator2/2
  Relational Operator2/1 -> Switch2/2
  [Efficiency] -> Product5/2, Product6/2
  Product5/1 -> Switch2/3
  Product6/1 -> Switch2/1
  Switch2/1 -> Subtract9/2, PowerElec_W/1  "Electric Power [W]"
  Subtract9/1 -> [PowerTh_W], PowerTherm_W/1  "Thermal Power [W]"
  1-D Lookup Table/1 -> [derate]
  dmw_kgps/1 -> [dmw_kgps]
  T_win_degC/1 -> [Twin_degC]
  [Twind_degC] -> 1-D Lookup Table/1
  Prelookup4/1 -> Motor EFFICIENCY MAP/3
  Prelookup4/2 -> Motor EFFICIENCY MAP/4
  Prelookup5/1 -> Motor EFFICIENCY MAP/5
  Prelookup5/2 -> Motor EFFICIENCY MAP/6
  Constant19/1 -> Motor EFFICIENCY MAP/7
  [Twind_degC] -> Prelookup5/1
  Constant9/1 -> Prelookup5/2
  Product/1 -> MaxTorque_Nm/1
  [derate] -> Product/1
  Subtract6/1 -> T_water_degC/1  "Water T [degC]"
  [Tsys0_degC] -> Discrete-Time Integrator1/2
  Product17/1 -> Discrete-Time Integrator1/1
  Product16/1 -> Product17/2
  [Tstat_degC] -> Subtract8/2
  Constant13/1 -> Product16/1
  Subtract8/1 -> Product18/1
  [Tsys0_degC] -> Delay1/2
  Constant16/1 -> Product16/2
  [Twin_degC] -> Subtract3/2
  Product8/1 -> Product9/1
  Product7/1 -> [tau]
  Product2/1 -> Product3/2
  [Tstat_degC] -> Subtract1/1
  Product1/1 -> Subtract1/2
  [Tsys0_degC] -> Discrete-Time Integrator/2
  Subtract4/1 -> Product10/2
  Constant12/1 -> Product2/1
  [Ptos_W] -> Subtract2/2
  [Ptow_W] -> Product1/2
  [PowerTh_W] -> Subtract2/1
  [Ptow_W] -> Subtract7/2
  Constant3/1 -> Product1/1
  Subtract1/1 -> Delay1/1
  Delay1/1 -> [Tbulk_degC]
  [cpw_JpkgpK] -> Product8/1
  Discrete-Time Integrator/1 -> [Twind_degC], T_windings_degC/1  "T_wind [degC]"
  Specific Heat Water-Glycol 80-20% vol [J/kgK]/1 -> [cpw_JpkgpK]
  Constant5/1 -> Product2/2
  Product9/1 -> Product10/1
  [Tbulk_degC] -> Specific Heat Water-Glycol 80-20% vol [J/kgK]/1
  Constant7/1 -> Product7/3
  Subtract3/1 -> Product9/2
  [cpw_JpkgpK] -> Product7/1
  Subtract2/1 -> Product3/1
  [Tstat_degC] -> Subtract3/1
  [dmw_kgps] -> Product8/2
  Product13/1 -> Subtract6/2
  Exp/1 -> Subtract4/2
  Product11/1 -> Exp/1
  [tau] -> Product12/2
  [Twin_degC] -> Subtract5/2
  Subtract5/1 -> Product13/1
  [Tstat_degC] -> Subtract6/1
  Product10/1 -> [Ptow_W]
  [tau] -> Product11/2
  [Tstat_degC] -> Subtract5/1
  Product12/1 -> Exp1/1
  Product18/1 -> [Ptos_W]
  [dmw_kgps] -> Product7/2
  Subtract7/1 -> Product17/1
  Constant4/1 -> Subtract4/1
  [Twind_degC] -> Subtract8/1
  Constant6/1 -> Product11/1
  [Ptos_W] -> Subtract7/1
  Constant8/1 -> Product12/1
  Exp1/1 -> Product13/2
  Constant20/1 -> Product18/2
  Product3/1 -> Discrete-Time Integrator/1
  Discrete-Time Integrator1/1 -> [Tstat_degC]  "T_stat [degC]"
  Bias/1 -> Product14/1
  Product14/1 -> Bias1/1
  Bias1/1 -> [Efficiency], Efficiency/1  "Efficiency"
  [Voltage_V] -> VoltageDependency/1
  VoltageDependency/1 -> Product14/2

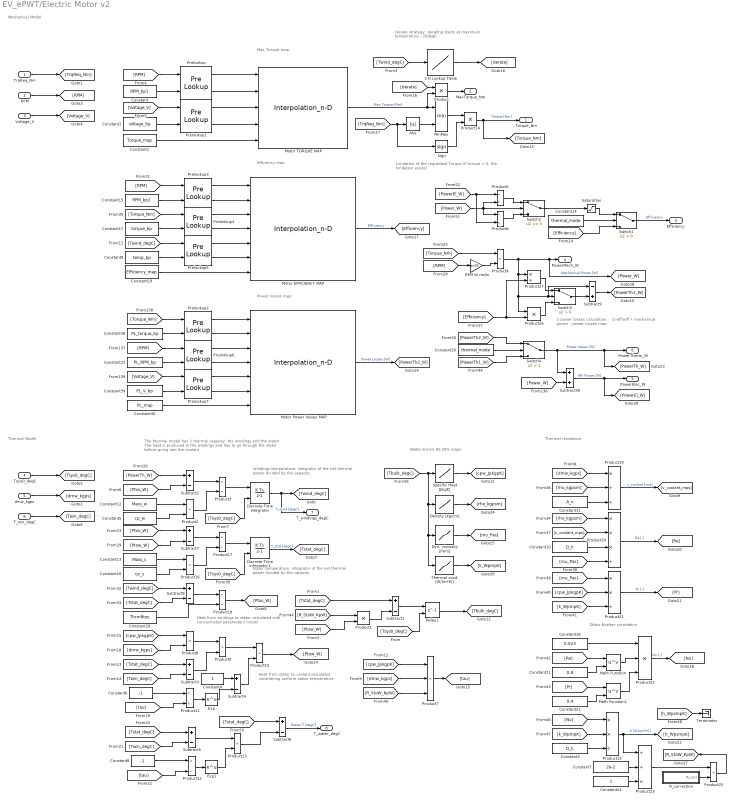
== system EV_ePWT/Electric Motor v2 ==
  note: Heat from stator to coolant calculated considering uniform stator temperature.
  note: Heat from windings to stator calculated with concentrated parameters model
  note: Stator temperature: integrator of the net thermal power divided by the capacity
  note: Windings temperature: integrator of the net thermal power divided by the capacity
  note: The thermal model has 2 thermal capacity: the windings and the stator. The heat is produced in the windings and has to go through the stator before going into the coolant
  note: Water-Glycol 80-20% maps
  note: Limitation of the requested Torque (if torque < 0, the limitation works)
  note: Derate strategy: derating starts at maximum temperature - 20degC
  note: Efficiency map
  note: Max Torque map
  note: Thermal Model
  note: Mechanical Model
  note: Thermal resistance
  note: Dittus-Boelter correlation
  note: Power losses map
  note: 2 power losses calculation:
      | - (1-eff)/eff * mechanical power
      | - power losses map
  TrqReq_Nm : Inport
  RPM : Inport  Port=2
  Voltage_V : Inport  Port=3
  Tsys0_degC : Inport  Port=4
  dmw_kgps : Inport  Port=5
  T_win_degC : Inport  Port=6
  1-D Lookup Table : Lookup_n-D  NumberOfTableDimensions=1  BreakpointsForDimension1=[-20 80 (MaxT-20) MaxT]  Table=[1 1 1 0]  InternalRulePriority=Speed  RndMeth=Simplest  InputSameDT=on
  Abs : Abs
  Constant : Constant  Value=RPM_bp1
  Constant1 : Constant  Value=voltage_bp
  Constant10 : Constant  Value=D_h
  Constant11 : Constant  Value=A_n
  Constant12 : Constant  Value=Mass_w
  Constant13 : Constant  Value=Mass_s
  Constant14 : Constant  Value=thermal_mode
  Constant15 : Constant  Value=RPM_bp2
  Constant16 : Constant  Value=cp_s
  Constant17 : Constant  Value=torque_bp
  Constant18 : Constant  Value=0.023
  Constant19 : Constant  Value=Efficiency_map
  Constant2 : Constant  Value=Torque_map
  Constant20 : Constant  Value=ThrmRtos
  Constant21 : Constant  Value=0.8
  Constant22 : Constant  Value=0.4
  Constant23 : Constant  Value=PL_RPM_bp
  Constant24 : Constant
  Constant26 : Constant  Value=thermal_mode
  Constant3 : Constant  Value=D_h
  Constant38 : Constant  Value=PL_torque_bp
  Constant39 : Constant  Value=PL_V_bp
  Constant4 : Constant
  Constant40 : Constant  Value=PL_map
  Constant5 : Constant  Value=cp_w
  Constant6 : Constant  Value=-1
  Constant7 : Constant  Value=2e-2
  Constant8 : Constant  Value=-1
  Constant9 : Constant  Value=temp_bp
  Delay1 : Delay  DelayLength=1  InitialConditionSource=Input port
      settings: InputPortMap=u0,p4
  Density [kg/cm] : Lookup_n-D  NumberOfTableDimensions=1  BreakpointsForDimension1=[-45.56 -17.78 10 37.77 65.55 93.33 121.11 148.88 176.66]  Table=[1020,1030,1030,1020,999,985,963,938,911]  ExtrapMethod=Clip  RndMeth=Simplest  InputSameDT=on
  Discrete-Time Integrator : DiscreteIntegrator  InitialConditionSource=external  SampleTime=-1  ICPrevOutput=DiscIntNeverNeededParam  ICPrevScaledInput=DiscIntNeverNeededParam
  Discrete-Time Integrator1 : DiscreteIntegrator  InitialConditionSource=external  SampleTime=-1  ICPrevOutput=DiscIntNeverNeededParam  ICPrevScaledInput=DiscIntNeverNeededParam
  Dyn. viscosity [Pa*s] : Lookup_n-D  NumberOfTableDimensions=1  BreakpointsForDimension1=[-45.56 -17.78 10 37.77 65.55 93.33 121.11 148.88 176.66]  Table=[640.26859,77.622,21.382,10.4477,6.2445,4.2234,3.1074,2.4377,1.98204]*1e-04  ExtrapMethod=Clip  RndMeth=Simplest  InputSameDT=on
  Exp : Math  SignedPower=off  SaturateOnIntegerOverflow=on
  Exp1 : Math  SignedPower=off  SaturateOnIntegerOverflow=on
  Math Function : Math  Operator=pow  SaturateOnIntegerOverflow=on
  Math Function1 : Math  Operator=pow  SaturateOnIntegerOverflow=on
  MinMax : MinMax  Inputs=2
  Motor EFFICIENCY MAP : Interpolation_n-D  NumberOfTableDimensions=3  TableSource=Input port
      settings: InputPortMap=u0,u1,u2,u3,u4,u5,p2
  Motor Power losses MAP : Interpolation_n-D  NumberOfTableDimensions=3  TableSource=Input port
      settings: InputPortMap=u0,u1,u2,u3,u4,u5,p2
  Motor TORQUE MAP : Interpolation_n-D  TableSource=Input port
      settings: InputPortMap=u0,u1,u2,u3,p2
  Prelookup{,1..7} (8 alike) : PreLookup  BreakpointsDataSource=Input port  BreakpointsData=[1:4]  FractionDataTypeStr=double
      settings: InputPortMap=u0,p1
  Product{,1..2,8..10,13..14,16,26} (10 alike) : Product
  Product{3,11..12,17..18,27} (6 alike) : Product  Inputs=*/
  Product15 : Product  Inputs=**/
  Product19 : Product  Inputs=*//
  Product20 : Product  Inputs=***/
  Product21 : Product  Inputs=**/
  Product22 : Product  Inputs=***
  Product23 : Product  Inputs=//*
  Product25 : Product  Inputs=**
  Product4 : Product  Inputs=**
  Product5 : Product  Inputs=/*
  Product6 : Product  Inputs=/*
  Product7 : Product  Inputs=3
  RPM to rad/s : Gain  Gain=pi/30
  R_correction : Subsystem  mask(Thermal resistance correction){}
      mask help:
      | The block outputs a value of correction (to be multiplied) for the thermal resistance [K/W].
      | It is calculated as the reference thermal resistance @lpm_ref @23degC divided by the target thermal resistance.
  Saturation : Saturate  UpperLimit=1  LowerLimit=0.5
  Sign : Signum
  Specific Heat [J/kgK] : Lookup_n-D  NumberOfTableDimensions=1  BreakpointsForDimension1=[-45.56 -17.78 10 37.77 65.55 93.33 121.11 148.88 176.66]  Table=[3841.6,3888.1,3934.6,3981.1,4027.6,4074.0,4120.5,4167.0,4213.6]  ExtrapMethod=Clip  RndMeth=Simplest  InputSameDT=on
  Subtract{1..8} (8 alike) : Sum  Inputs=+-
  Subtract38 : Sum
  Subtract9 : Sum  Inputs=-+
  Switch1 : Switch  Criteria=u2 > Threshold
  Switch2 : Switch
  Switch3 : Switch  Criteria=u2 > Threshold
  Switch4 : Switch  Criteria=u2 > Threshold  Threshold=1
  Terminator : Terminator
  Thermal cond. [W/(m*K)] : Lookup_n-D  NumberOfTableDimensions=1  BreakpointsForDimension1=[-45.56 -17.78 10 37.77 65.55 93.33 121.11 148.88 176.66]  Table=[0.433474,0.474305,0.507306,0.532476,0.549815,0.559304,0.561011,0.554885,0.540929]  ExtrapMethod=Clip  RndMeth=Simplest  InputSameDT=on
  Torque_Nm : Outport
  MaxTorque_Nm : Outport  Port=2
  Efficiency : Outport  Port=3
  PowerMech_W : Outport  Port=4
  PowerElec_W : Outport  Port=5
  PowerTherm_W : Outport  Port=6
  T_windings_degC : Outport  Port=7
  T_water_degC : Outport  Port=8
  wires:
  Motor EFFICIENCY MAP/1 -> [Efficiency]  "Efficiency"
  Discrete-Time Integrator1/1 -> [Tstat_degC]  "T_stat [degC]"
  Product3/1 -> Discrete-Time Integrator/1
  Constant20/1 -> Product18/2
  Exp1/1 -> Product13/2
  Constant8/1 -> Product12/1
  [Ptos_W] -> Subtract7/1
  Constant6/1 -> Product11/1
  [Twind_degC] -> Subtract8/1
  Constant4/1 -> Subtract4/1
  Subtract7/1 -> Product17/1
  [dmw_kgps] -> Product7/2
  Product18/1 -> [Ptos_W]
  Product12/1 -> Exp1/1
  [Tstat_degC] -> Subtract5/1
  [tau] -> Product11/2
  Product10/1 -> [Ptow_W]
  [Tstat_degC] -> Subtract6/1
  Subtract5/1 -> Product13/1
  [Twin_degC] -> Subtract5/2
  [tau] -> Product12/2
  Product11/1 -> Exp/1
  Exp/1 -> Subtract4/2
  Product13/1 -> Subtract6/2
  [dmw_kgps] -> Product8/2
  [Tstat_degC] -> Subtract3/1
  Subtract2/1 -> Product3/1
  [cpw_JpkgpK] -> Product7/1
  Subtract3/1 -> Product9/2
  [R_StoW_KpW] -> Product7/3
  Product9/1 -> Product10/1
  Constant5/1 -> Product2/2
  Discrete-Time Integrator/1 -> T_windings_degC/1, [Twind_degC]  "T_wind [degC]"
  [cpw_JpkgpK] -> Product8/1
  Delay1/1 -> [Tbulk_degC]
  Subtract1/1 -> Delay1/1
  [R_StoW_KpW] -> Product1/1
  [Ptow_W] -> Subtract7/2
  [PowerTh_W] -> Subtract2/1
  [Ptow_W] -> Product1/2
  [Ptos_W] -> Subtract2/2
  Constant12/1 -> Product2/1
  Subtract4/1 -> Product10/2
  [Tsys0_degC] -> Discrete-Time Integrator/2
  Product1/1 -> Subtract1/2
  [Tstat_degC] -> Subtract1/1
  Product2/1 -> Product3/2
  Product7/1 -> [tau]
  Product8/1 -> Product9/1
  [Twin_degC] -> Subtract3/2
  Constant16/1 -> Product16/2
  [Tsys0_degC] -> Delay1/2
  Subtract8/1 -> Product18/1
  Constant13/1 -> Product16/1
  [Tstat_degC] -> Subtract8/2
  Product16/1 -> Product17/2
  Product17/1 -> Discrete-Time Integrator1/1
  [Tsys0_degC] -> Discrete-Time Integrator1/2
  Subtract6/1 -> T_water_degC/1  "Water T [degC]"
  [derate] -> Product/1
  Product/1 -> MaxTorque_Nm/1
  Constant9/1 -> Prelookup5/2
  [Twind_degC] -> Prelookup5/1
  Constant19/1 -> Motor EFFICIENCY MAP/7
  Prelookup5/2 -> Motor EFFICIENCY MAP/6
  Prelookup5/1 -> Motor EFFICIENCY MAP/5
  Prelookup4/2 -> Motor EFFICIENCY MAP/4
  Prelookup4/1 -> Motor EFFICIENCY MAP/3
  [Twind_degC] -> 1-D Lookup Table/1
  T_win_degC/1 -> [Twin_degC]
  dmw_kgps/1 -> [dmw_kgps]
  1-D Lookup Table/1 -> [derate]
  Product4/1 -> Subtract9/1, Switch3/2, Product26/1, Product27/1, [Power_W], PowerMech_W/1  "Mechanical Power [W]"
  RPM to rad/s/1 -> Product4/2
  [Torque_Nm] -> Product4/1
  [RPM] -> RPM to rad/s/1
  Constant17/1 -> Prelookup4/2
  [RPM] -> Prelookup3/1
  Prelookup3/1 -> Motor EFFICIENCY MAP/1
  [Torque_Nm] -> Prelookup4/1
  Prelookup3/2 -> Motor EFFICIENCY MAP/2
  Constant15/1 -> Prelookup3/2
  [TrqReq_Nm] -> Sign/1, Abs/1
  Motor TORQUE MAP/1 -> Product/2, MinMax/1  "Max Torque [Nm]"
  Constant2/1 -> Motor TORQUE MAP/5
  Constant/1 -> Prelookup/2
  TrqReq_Nm/1 -> [TrqReq_Nm]
  Prelookup/2 -> Motor TORQUE MAP/2
  Tsys0_degC/1 -> [Tsys0_degC]
  Voltage_V/1 -> [Voltage_V]
  RPM/1 -> [RPM]
  [Voltage_V] -> Prelookup1/1
  Prelookup/1 -> Motor TORQUE MAP/1
  [RPM] -> Prelookup/1
  Constant1/1 -> Prelookup1/2
  [Tbulk_degC] -> Density [kg/cm]/1, Thermal cond. [W/(m*K)]/1, Dyn. viscosity [Pa*s]/1, Specific Heat [J/kgK]/1
  Constant11/1 -> Product19/3
  [rho_kgpsm] -> Product19/2
  Product19/1 -> [v_coolant_mps]  "v_coolant [m/s]"
  [rho_kgpsm] -> Product20/1
  [v_coolant_mps] -> Product20/2
  Constant10/1 -> Product20/3
  [mu_Pas] -> Product20/4
  Product20/1 -> [Re]  "Re [-]"
  [mu_Pas] -> Product21/1
  [cpw_JpkgpK] -> Product21/2
  [k_WpmpK] -> Product21/3
  Product21/1 -> [Pr]  "Pr [-]"
  Constant18/1 -> Product22/1
  Math Function/1 -> Product22/2
  Math Function1/1 -> Product22/3
  Constant22/1 -> Math Function1/2
  Constant21/1 -> Math Function/2
  [Re] -> Math Function/1
  [Pr] -> Math Function1/1
  Product22/1 -> [Nu]  "Nu [-]"
  [Nu] -> Product15/1
  [k_WpmpK] -> Product15/2
  Constant3/1 -> Product15/3
  Product15/1 -> [h_WpsmpK], Product23/1  "h [W(sm*K)]"
  Constant7/1 -> Product23/2
  Constant24/1 -> Product23/3
  [h_WpsmpK] -> Terminator/1
  Specific Heat [J/kgK]/1 -> [cpw_JpkgpK]
  Density [kg/cm]/1 -> [rho_kgpsm]
  Dyn. viscosity [Pa*s]/1 -> [mu_Pas]
  Thermal cond. [W/(m*K)]/1 -> [k_WpmpK]
  Product23/1 -> Product25/1
  Product25/1 -> [R_StoW_KpW]
  [dmw_kgps] -> Product19/1
  R_correction/1(R_corr) -> Product25/2
  [Voltage_V] -> Prelookup7/1
  [Torque_Nm] -> Prelookup2/1
  Constant38/1 -> Prelookup2/2
  Constant39/1 -> Prelookup7/2
  [RPM] -> Prelookup6/1
  Constant23/1 -> Prelookup6/2
  Prelookup2/2 -> Motor Power losses MAP/2
  Prelookup2/1 -> Motor Power losses MAP/1
  Prelookup6/1 -> Motor Power losses MAP/3
  Prelookup6/2 -> Motor Power losses MAP/4
  Prelookup7/1 -> Motor Power losses MAP/5
  Prelookup7/2 -> Motor Power losses MAP/6
  Prelookup1/2 -> Motor TORQUE MAP/4
  Prelookup1/1 -> Motor TORQUE MAP/3
  Constant40/1 -> Motor Power losses MAP/7
  Abs/1 -> MinMax/2
  MinMax/1 -> Product14/1
  Sign/1 -> Product14/2
  Product14/1 -> [Torque_Nm], Torque_Nm/1  "Torque [Nm]"
  Motor Power losses MAP/1 -> [PowerTh2_W]  "Power Losses [W]"
  Constant26/1 -> Switch4/2
  Subtract9/1 -> [PowerTh1_W]
  [PowerTh1_W] -> Switch4/3
  [PowerTh2_W] -> Switch4/1
  [Efficiency] -> Product26/2, Product27/2
  Product27/1 -> Switch3/1
  Product26/1 -> Switch3/3
  Switch3/1 -> Subtract9/2
  Switch4/1 -> [PowerTh_W], PowerTherm_W/1, Subtract38/1  "Power losses [W]"
  Subtract38/1 -> [PowerEl_W], PowerElec_W/1  "INV Power [W]"
  [Power_W] -> Subtract38/2
  Constant14/1 -> Switch1/2
  [Efficiency] -> Switch1/3
  Switch1/1 -> Efficiency/1  "Efficiency"
  Switch2/1 -> Saturation/1
  [Power_W] -> Product6/1, Product5/2, Switch2/2
  Product5/1 -> Switch2/1
  Product6/1 -> Switch2/3
  [PowerEl_W] -> Product6/2, Product5/1
  Saturation/1 -> Switch1/1
